simulink model "mech_fceng1"  (Simulink 7.1)
settings: Solver=ode45  StartTime=0.0  StopTime=inf  RelTol=1e-3  AbsTol=1e-4
PreLoadFcn:
  | mech_fceng_init;load mech_fceng_images;
InitFcn:
  | mech_slider_open(gcs);
values from neighbouring files (symbols this model uses):
  AirRo = 1.2E-3    (= 0.0012)    [mech_sceng_init.m]
  Cv = 3    [mech_sceng_init.m]
  G = 9.81    [mech_motorcycle_data.m]    (also in mech_sceng_init.m = 1.4)
  Pa = 1033.34    [mech_sceng_init.m]
  Q = 46816    [mech_sceng_init.m]
  R = y([30:p],2)./y([30:p],1)    [mech_car_handling_sweep.m]    (also in mech_flexible_beamelement.m = [1  0  0; mech_sceng_init.m = 5; mech_toroid_setup.m = 10)
  Ta = 25    [mech_sceng_init.m]
  Vo = pi*R*R*14    (= 1099.55742876)    [mech_sceng_init.m]
  Vtdc = pi*R*R*2    (= 157.079632679)    [mech_sceng_init.m]
libraries: mblibv1 x47, simulink x3, simulink_extras x1
(part 1 of 2)
settings Model: Creator=The MathWorks Inc.  LastModifiedBy=Administrator  ExtModeAutoUpdateStatusClock=off
settings DataIOCC: SignalLoggingName=sigsOut
settings OptimizationCC: BooleanDataType=off  InlineInvariantSignals=on  BufferReusableBoundary=off
settings DebuggingCC: SaveWithParameterizedLinksMsg=none  CheckExecutionContextPreStartOutputMsg=on  CheckExecutionContextRuntimeOutputMsg=on  SignalResolutionControl=TryResolveAllWithWarning  SolverPrmCheckMsg=none  MultiTaskDSMMsg=warning  MultiTaskCondExecSysMsg=none  SigSpecEnsureSampleTimeMsg=none  UnconnectedInputMsg=none  UnconnectedOutputMsg=none  UnconnectedLineMsg=none  StrictBusMsg=None
settings HardwareCC: ProdHWDeviceType=Specified  TargetEndianess=LittleEndian  TargetHWDeviceType=MATLAB Host  ProdEqTarget=off
settings RTWCC: SystemTargetFile=rsim.tlc  TemplateMakefile=rsim_default_tmf  Description=Rapid Simulation Target  ProcessScript=rsim_make_rtw_hook  IncludeERTFirstTime=on
settings RSimTargetCC: TargetFcnLib=ansi_tfl_tmw.mat  TargetFunctionLibrary=ANSI_C  IsPILTarget=off  EnableShiftOperators=on  PortableWordSizes=off
settings SimMechanicsCC: WarnOnRedundantConstraints=off

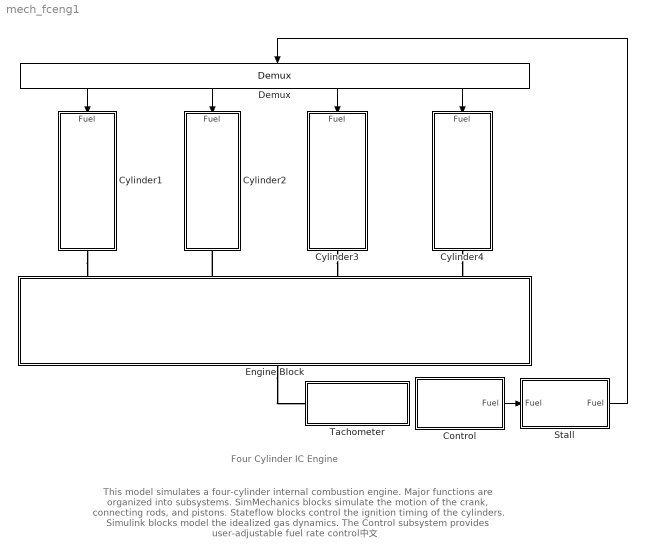
== system mech_fceng1 ==
  note: This model simulates a four-cylinder internal combustion engine. Major functions are organized into subsystems. SimMechanics blocks simulate the motion of the crank, connecting rods, and pistons. Stateflow blocks control the ignition timing of the cylinders. Simulink blocks model the idealized gas dynamics. The Control subsystem provides user-adjustable fuel rate control.中文
  note: Four Cylinder IC Engine
  Control : Subsystem  Tag=OpenMeAtStartUp
  Cylinder1 : Subsystem  Orientation=down
      mask Display: image(crodassm);
  Cylinder2 : Subsystem  Orientation=down
      mask Display: image(crodassmb);
  Cylinder3 : Subsystem  Orientation=down
      mask Display: image(crodassmb);
  Cylinder4 : Subsystem  Orientation=down
      mask Display: image(crodassm);
  Demux : Demux  Orientation=down
  Engine Block : Subsystem  Orientation=up
      mask Display: image(crank);
  Stall : Subsystem
  Tachometer : Subsystem
  wires:
  Demux/1 -> Cylinder1/1(Fuel)
  Demux/2 -> Cylinder2/1(Fuel)
  Demux/3 -> Cylinder3/1(Fuel)
  Demux/4 -> Cylinder4/1(Fuel)
  Control/1(Fuel) -> Stall/1("Fuel ")
  Stall/1(Fuel) -> Demux/1
  connections:
  Cylinder1/RConn1 -- Engine Block/RConn1
  Cylinder4/RConn1 -- Engine Block/RConn4
  Engine Block/LConn1 -- Tachometer/LConn1
  Cylinder3/RConn1 -- Engine Block/RConn3
  Engine Block/RConn2 -- Cylinder2/RConn1

== system mech_fceng1/Control ==
  Constant : Constant  OutDataType=sfix(16)  OutScaling=2^0
  Cylinder1 : simulink/Signal Routing/Manual Switch  Orientation=down  SystemSampleTime=-1  sw=0  action=0  varsize=off
  Cylinder4 : simulink/Signal Routing/Manual Switch  Orientation=down  SystemSampleTime=-1  sw=0  action=0  varsize=off
  Fuel Control : simulink/Math Operations/Slider Gain  Tag="674   438   332   100"  SystemSampleTime=-1  low=0  gain=2  high=4
  OFF : Constant  Orientation=up  Value=0  OutDataType=sfix(16)  OutScaling=2^0
  ON : Constant  Orientation=up  Value=-1  OutDataType=sfix(16)  OutScaling=2^0
  Fuel : Outport  OutDataType=sfix(16)  OutScaling=2^0
  tag scope: Cylinder1=global, Cylinder2=global
  wires:
  Cylinder1/1 -> [Cylinder1]
  Constant/1 -> Fuel Control/1
  Fuel Control/1 -> Fuel/1
  OFF/1 -> Cylinder1/1, Cylinder4/1
  ON/1 -> Cylinder4/2, Cylinder1/2
  Cylinder4/1 -> [Cylinder2]

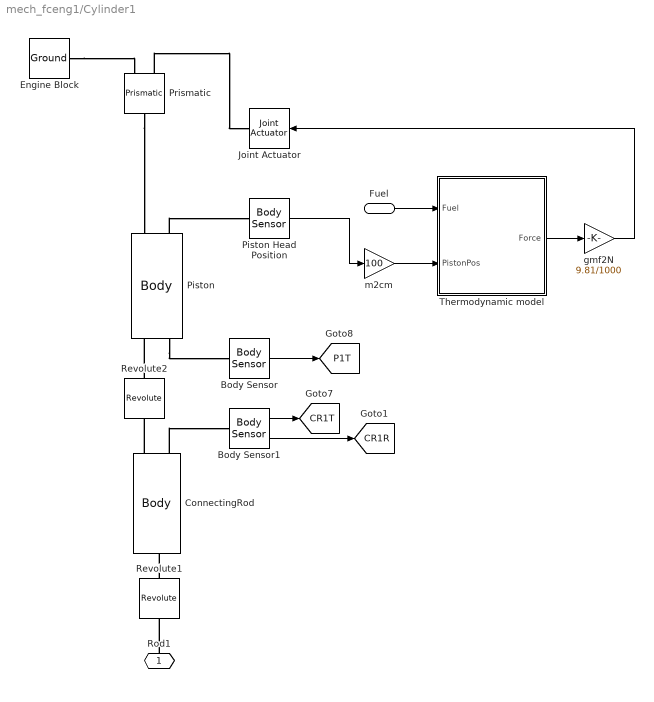
== system mech_fceng1/Cylinder1 ==
  Fuel : Inport  OutDataType=sfix(16)  OutScaling=2^0
  Body Sensor : mblibv1/Sensors &  Actuators/Body Sensor  DialogController=MECH.DynMechDlgSource  SystemSampleTime=-1  PhysicalDomain=Mechanical  PortType=blob  Muxed=on  Pose=off  Angle=on  AngleUnits=deg  ArcVelocity=off  ArcVelocityUnits=deg/s  ArcAcceleration=off  ArcAccelerationUnits=deg/s^2  CoordPosition=on  CoordPositionUnits=m  Velocity=off  VelocityUnits=m/s  Acceleration=off  AccelerationUnits=m/s^2  Quaternion=on  QuaternionDT=off  QuaternionDDT=off  QuaternionUnits=off  OutputVector=[1]  ActiveIO=on  Width=3  DialogClass=MechanicalSensorBlock  ReferenceFrame=Absolute (World)
  Body Sensor1 : mblibv1/Sensors &  Actuators/Body Sensor  DialogController=MECH.DynMechDlgSource  SystemSampleTime=-1  PhysicalDomain=Mechanical  PortType=blob  Muxed=off  Pose=on  Angle=on  AngleUnits=deg  ArcVelocity=off  ArcVelocityUnits=deg/s  ArcAcceleration=off  ArcAccelerationUnits=deg/s^2  CoordPosition=on  CoordPositionUnits=m  Velocity=off  VelocityUnits=m/s  Acceleration=off  AccelerationUnits=m/s^2  Quaternion=on  QuaternionDT=off  QuaternionDDT=off  QuaternionUnits=off  OutputVector=[ 3 9 ]  ActiveIO=on  Width=12  DialogClass=MechanicalSensorBlock  ReferenceFrame=Absolute (World)
  ConnectingRod : mblibv1/Bodies/Body  Orientation=up  DialogController=MECH.DynMechDlgSource  PhysicalDomain=mechanical  SubClassName=Unknown  LeftPortType=workingframe  RightPortType=workingframe  LConnTagsString=CS1  RConnTagsString=CS2|CS3  DialogClass=MechanicalBodyBlock  Mass=676.73  MassUnits=g  InertiaUnits=kg*m^2  Inertia=[37007.64 0 -0.01;0 2936.99 7181.27;-0.01 7181.27 34460.53]*1E-7  Shape=Cylinder  ShapeDims=[1 1]  ShapeUnits=m  ShapeUse=false  Density=1  DensityUnits=kg/m^3  DensityUse=false  GraphicsMode=1  BodyColor=[0.5 0.5 0.5]  GraphicsObj=[]  AttachedToCS=1  CG=Left$CG$[-18 11.35 -2.70]$WORLD$WORLD$cm$[0 0 0]$Euler X-Y-Z$deg$WORLD$false  WorkingFrames=Left$CS1$[-18 4.24 -4.24]$WORLD$WORLD$cm$[0 0 0]$Euler X-Y-Z$deg$WORLD$true#Right$CS2$[-18 23.79 0]$WORLD$WORLD$cm$[0 0 0]$Euler X-Y-Z$deg$WORLD$true#Right$CS3$[-18 4.24 -4.24]$WORLD$WORLD$cm$[0 0 0]$Euler X-Y-Z$deg$WORLD$true  CGPos=[-18 11.35 -2.70]  CGRot=[0 0 0]  CS0Pos=[]  CS0Rot=[]  CS1Pos=[-18 4.24 -4.24]  CS1Rot=[0 0 0]  CS2Pos=[-18 23.79 0]  CS2Rot=[0 0 0]  CS3Pos=[-18 4.24 -4.24]  CS3Rot=[0 0 0]  CS4Pos=[]  CS4Rot=[]  CS5Pos=[]  CS5Rot=[]  CS6Pos=[]  CS6Rot=[]  CS7Pos=[]  CS7Rot=[]  CS8Pos=[]  CS8Rot=[]  CS9Pos=[]  CS9Rot=[]  CS10Pos=[]  CS10Rot=[]  CS11Pos=[]  CS11Rot=[]  CS12Pos=[]  CS12Rot=[]  CS13Pos=[]  CS13Rot=[]  CS14Pos=[]  CS14Rot=[]  CS15Pos=[]  CS15Rot=[]  CS16Pos=[]  CS16Rot=[]  CS17Pos=[]  CS17Rot=[]  CS18Pos=[]  CS18Rot=[]  CS19Pos=[]  CS19Rot=[]  CS20Pos=[]  CS20Rot=[]
  Engine Block : mblibv1/Bodies/Ground  DialogController=MECH.DynMechDlgSource  SystemSampleTime=-1  LeftPortType=env  RightPortType=workingframe  PhysicalDomain=Mechanical  DialogClass=GroundBlock  CoordPosition=[-13.23 23.79 0]  CoordPositionUnits=cm  StateVectorMgrId=-1  MachineId=[0 0]  ShowEnvPort=off
  Joint Actuator : mblibv1/Sensors &  Actuators/Joint Actuator  Orientation=left  DialogController=MECH.DynMechDlgSource  SystemSampleTime=-1  PhysicalDomain=Mechanical  PortType=blob  ActuationStyle=Force  AngleUnits=deg  ArcVelocityUnits=deg/s  ArcAccelerationUnits=deg/s^2  CoordPositionUnits=m  VelocityUnits=m/s  AccelerationUnits=m/s^2  ForceUnits=N  TorqueUnits=N-m  ActiveIO=on  Width=1  DialogClass=MechanicalActuatorBlock  Primitive=P1  ReferenceFrame=Absolute (INERTIAL)
  Piston : mblibv1/Bodies/Body  Orientation=up  DialogController=MECH.DynMechDlgSource  PhysicalDomain=mechanical  SubClassName=Unknown  LeftPortType=workingframe  RightPortType=workingframe  LConnTagsString=CS1|CS3  RConnTagsString=CS2|CS4  DialogClass=MechanicalBodyBlock  Mass=3490.25  MassUnits=g  InertiaUnits=kg*m^2  Inertia=[39798.30 0.06 -0.01;0.06 49173.25 -0.04;-0.01 -0.04 39108.48]*1E-7  Shape=Cylinder  ShapeDims=[1 1]  ShapeUnits=m  ShapeUse=false  Density=1  DensityUnits=kg/m^3  DensityUse=false  GraphicsMode=1  BodyColor=[0.5 0.5 0.5]  GraphicsObj=[]  AttachedToCS=1  CG=Left$CG$[-18 24.51 0]$WORLD$WORLD$cm$[0 0 0]$Euler X-Y-Z$deg$WORLD$false  WorkingFrames=Left$CS1$[-18 23.79 0]$WORLD$WORLD$cm$[0 0 0]$Euler X-Y-Z$deg$WORLD$true#Right$CS2$[-13.23 23.79 0]$WORLD$WORLD$cm$[0 0 0]$Euler X-Y-Z$deg$WORLD$true#Left$CS3$[-18 23.79 0]$WORLD$WORLD$cm$[0 0 0]$Euler X-Y-Z$deg$WORLD$true#Right$CS4$[-18 23.79+4 0]$WORLD$WORLD$cm$[0 0 0]$Euler X-Y-Z$deg$WORLD$true  CGPos=[-18 24.51 0]  CGRot=[0 0 0]  CS0Pos=[]  CS0Rot=[]  CS1Pos=[-18 23.79 0]  CS1Rot=[0 0 0]  CS2Pos=[-13.23 23.79 0]  CS2Rot=[0 0 0]  CS3Pos=[-18 23.79 0]  CS3Rot=[0 0 0]  CS4Pos=[-18 23.79+4 0]  CS4Rot=[0 0 0]  CS5Pos=[]  CS5Rot=[]  CS6Pos=[]  CS6Rot=[]  CS7Pos=[]  CS7Rot=[]  CS8Pos=[]  CS8Rot=[]  CS9Pos=[]  CS9Rot=[]  CS10Pos=[]  CS10Rot=[]  CS11Pos=[]  CS11Rot=[]  CS12Pos=[]  CS12Rot=[]  CS13Pos=[]  CS13Rot=[]  CS14Pos=[]  CS14Rot=[]  CS15Pos=[]  CS15Rot=[]  CS16Pos=[]  CS16Rot=[]  CS17Pos=[]  CS17Rot=[]  CS18Pos=[]  CS18Rot=[]  CS19Pos=[]  CS19Rot=[]  CS20Pos=[]  CS20Rot=[]
  Piston Head Position : mblibv1/Sensors &  Actuators/Body Sensor  DialogController=MECH.DynMechDlgSource  SystemSampleTime=-1  PhysicalDomain=Mechanical  PortType=blob  Muxed=on  Pose=off  Angle=on  AngleUnits=deg  ArcVelocity=off  ArcVelocityUnits=deg/s  ArcAcceleration=off  ArcAccelerationUnits=deg/s^2  CoordPosition=on  CoordPositionUnits=m  Velocity=off  VelocityUnits=m/s  Acceleration=off  AccelerationUnits=m/s^2  Quaternion=on  QuaternionDT=off  QuaternionDDT=off  QuaternionUnits=off  OutputVector=[1]  ActiveIO=on  Width=3  DialogClass=MechanicalSensorBlock  ReferenceFrame=Absolute (World)
  Prismatic : mblibv1/Joints/Prismatic  Orientation=down  DialogController=MECH.DynMechDlgSource  PhysicalDomain=mechanical  SubClassName=Unknown  LeftPortType=blob  RightPortType=blob  LConnTagsString=__newl0|SA1  RConnTagsString=__newr0  NumSAPorts=1  CutJoint=off  MarkAsCut=off  Primitives=prismatic  PrimitiveProps=P1$WORLD$[0 1 0]$prismatic  DialogClass=JointBlock  P1Axis=[0 1 0]
  Revolute1 : mblibv1/Joints/Revolute  Orientation=up  DialogController=MECH.DynMechDlgSource  PhysicalDomain=mechanical  SubClassName=Unknown  LeftPortType=blob  RightPortType=blob  LConnTagsString=__newl0  RConnTagsString=__newr0  NumSAPorts=0  CutJoint=off  MarkAsCut=off  Primitives=revolute  PrimitiveProps=R1$WORLD$[1 0 0]$revolute  DialogClass=JointBlock  R1Axis=[1 0 0]
  Revolute2 : mblibv1/Joints/Revolute  Orientation=up  DialogController=MECH.DynMechDlgSource  PhysicalDomain=mechanical  SubClassName=Unknown  LeftPortType=blob  RightPortType=blob  LConnTagsString=__newl0  RConnTagsString=__newr0  NumSAPorts=0  CutJoint=on  MarkAsCut=off  Primitives=revolute  PrimitiveProps=R1$WORLD$[1 0 0]$revolute  DialogClass=JointBlock  R1Axis=[1 0 0]
  Thermodynamic model : Subsystem
  gmf2N : Gain  Gain=9.81/1000  ParameterDataType=sfix(16)  ParameterScaling=2^0  OutDataType=sfix(16)  OutScaling=2^0  SaturateOnIntegerOverflow=on  OutDataTypeStr=Inherit: Same as input  ParamDataTypeStr=Inherit: Same as input
  m2cm : Gain  Gain=100  ParameterDataType=sfix(16)  ParameterScaling=2^0  OutDataType=sfix(16)  OutScaling=2^0  SaturateOnIntegerOverflow=on  OutDataTypeStr=Inherit: Same as input  ParamDataTypeStr=Inherit: Same as input
  Rod1 : PMIOPort  Orientation=up  Port=1  Side=Right
  tag scope: CR1R=global, CR1T=global, P1T=global
  wires:
  Body Sensor1/2 -> [CR1R]
  Body Sensor1/1 -> [CR1T]
  Body Sensor/1 -> [P1T]
  gmf2N/1 -> Joint Actuator/1
  Fuel/1 -> Thermodynamic model/1(Fuel)
  Piston Head Position/1 -> m2cm/1
  Thermodynamic model/1(Force) -> gmf2N/1
  m2cm/1 -> Thermodynamic model/2(PistonPos)
  connections:
  Prismatic/LConn2 -- Joint Actuator/RConn1
  Prismatic/RConn1 -- Piston/RConn1
  Engine Block/RConn1 -- Prismatic/LConn1
  ConnectingRod/RConn2 -- Body Sensor1/LConn1
  Piston/LConn2 -- Body Sensor/LConn1
  Piston/RConn2 -- Piston Head Position/LConn1
  Rod1/RConn1 -- Revolute1/LConn1
  Revolute2/RConn1 -- Piston/LConn1
  ConnectingRod/RConn1 -- Revolute2/LConn1
  Revolute1/RConn1 -- ConnectingRod/LConn1

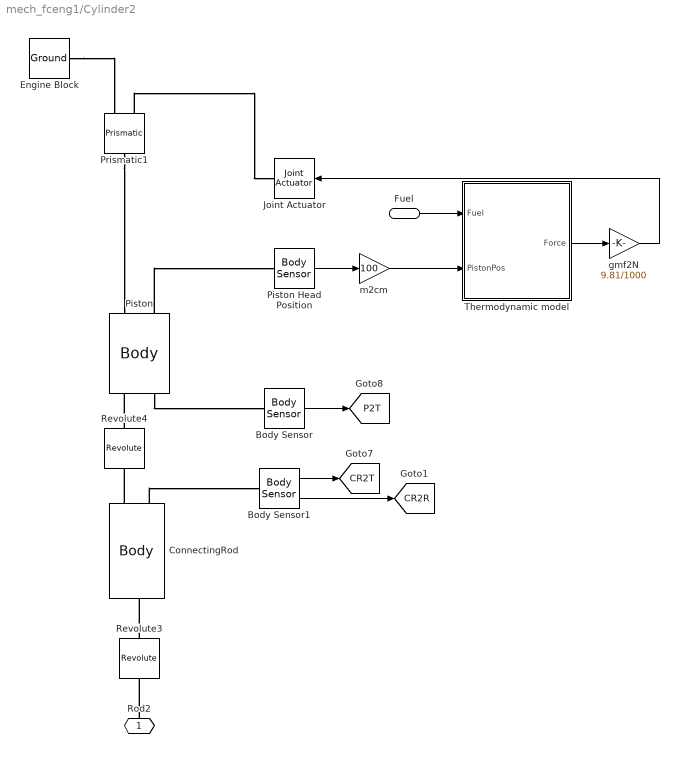
== system mech_fceng1/Cylinder2 ==
  Fuel : Inport  OutDataType=sfix(16)  OutScaling=2^0
  Body Sensor : mblibv1/Sensors &  Actuators/Body Sensor  DialogController=MECH.DynMechDlgSource  SystemSampleTime=-1  PhysicalDomain=Mechanical  PortType=blob  Muxed=on  Pose=off  Angle=on  AngleUnits=deg  ArcVelocity=off  ArcVelocityUnits=deg/s  ArcAcceleration=off  ArcAccelerationUnits=deg/s^2  CoordPosition=on  CoordPositionUnits=m  Velocity=off  VelocityUnits=m/s  Acceleration=off  AccelerationUnits=m/s^2  Quaternion=on  QuaternionDT=off  QuaternionDDT=off  QuaternionUnits=off  OutputVector=[1]  ActiveIO=on  Width=3  DialogClass=MechanicalSensorBlock  ReferenceFrame=Absolute (World)
  Body Sensor1 : mblibv1/Sensors &  Actuators/Body Sensor  DialogController=MECH.DynMechDlgSource  SystemSampleTime=-1  PhysicalDomain=Mechanical  PortType=blob  Muxed=off  Pose=on  Angle=on  AngleUnits=deg  ArcVelocity=off  ArcVelocityUnits=deg/s  ArcAcceleration=off  ArcAccelerationUnits=deg/s^2  CoordPosition=on  CoordPositionUnits=m  Velocity=off  VelocityUnits=m/s  Acceleration=off  AccelerationUnits=m/s^2  Quaternion=on  QuaternionDT=off  QuaternionDDT=off  QuaternionUnits=off  OutputVector=[ 3 9 ]  ActiveIO=on  Width=12  DialogClass=MechanicalSensorBlock  ReferenceFrame=Absolute (World)
  ConnectingRod : mblibv1/Bodies/Body  Orientation=up  DialogController=MECH.DynMechDlgSource  PhysicalDomain=mechanical  SubClassName=Unknown  LeftPortType=workingframe  RightPortType=workingframe  LConnTagsString=CS1  RConnTagsString=CS2|CS3  DialogClass=MechanicalBodyBlock  Mass=676.73  MassUnits=g  InertiaUnits=kg*m^2  Inertia=[37007.64 0 -0.01;0 2936.99 7181.27;-0.01 7181.27 34460.53]*1E-7  Shape=Cylinder  ShapeDims=[1 1]  ShapeUnits=m  ShapeUse=false  Density=1  DensityUnits=kg/m^3  DensityUse=false  GraphicsMode=1  BodyColor=[0.5 0.5 0.5]  GraphicsObj=[]  AttachedToCS=1  CG=Left$CG$[-6 2.87 2.70]$WORLD$WORLD$cm$[0 0 0]$Euler X-Y-Z$deg$WORLD$false  WorkingFrames=Left$CS1$[-6 -4.24 4.24]$WORLD$WORLD$cm$[0 0 0]$Euler X-Y-Z$deg$WORLD$true#Right$CS2$[-6 15.30 0]$WORLD$WORLD$cm$[0 0 0]$Euler X-Y-Z$deg$WORLD$true#Right$CS3$[-6 -4.24 4.24]$WORLD$WORLD$cm$[0 0 0]$Euler X-Y-Z$deg$WORLD$true  CGPos=[-6 2.87 2.70]  CGRot=[0 0 0]  CS0Pos=[]  CS0Rot=[]  CS1Pos=[-6 -4.24 4.24]  CS1Rot=[0 0 0]  CS2Pos=[-6 15.30 0]  CS2Rot=[0 0 0]  CS3Pos=[-6 -4.24 4.24]  CS3Rot=[0 0 0]  CS4Pos=[]  CS4Rot=[]  CS5Pos=[]  CS5Rot=[]  CS6Pos=[]  CS6Rot=[]  CS7Pos=[]  CS7Rot=[]  CS8Pos=[]  CS8Rot=[]  CS9Pos=[]  CS9Rot=[]  CS10Pos=[]  CS10Rot=[]  CS11Pos=[]  CS11Rot=[]  CS12Pos=[]  CS12Rot=[]  CS13Pos=[]  CS13Rot=[]  CS14Pos=[]  CS14Rot=[]  CS15Pos=[]  CS15Rot=[]  CS16Pos=[]  CS16Rot=[]  CS17Pos=[]  CS17Rot=[]  CS18Pos=[]  CS18Rot=[]  CS19Pos=[]  CS19Rot=[]  CS20Pos=[]  CS20Rot=[]
  Engine Block : mblibv1/Bodies/Ground  DialogController=MECH.DynMechDlgSource  SystemSampleTime=-1  LeftPortType=env  RightPortType=workingframe  PhysicalDomain=Mechanical  DialogClass=GroundBlock  CoordPosition=[-1 15.30 0]  CoordPositionUnits=cm  StateVectorMgrId=-1  MachineId=[0 0]  ShowEnvPort=off
  Joint Actuator : mblibv1/Sensors &  Actuators/Joint Actuator  Orientation=left  DialogController=MECH.DynMechDlgSource  SystemSampleTime=-1  PhysicalDomain=Mechanical  PortType=blob  ActuationStyle=Force  AngleUnits=deg  ArcVelocityUnits=deg/s  ArcAccelerationUnits=deg/s^2  CoordPositionUnits=m  VelocityUnits=m/s  AccelerationUnits=m/s^2  ForceUnits=N  TorqueUnits=N-m  ActiveIO=on  Width=1  DialogClass=MechanicalActuatorBlock  Primitive=P1  ReferenceFrame=Absolute (INERTIAL)
  Piston : mblibv1/Bodies/Body  Orientation=up  DialogController=MECH.DynMechDlgSource  PhysicalDomain=mechanical  SubClassName=Unknown  LeftPortType=workingframe  RightPortType=workingframe  LConnTagsString=CS1|CS3  RConnTagsString=CS2|CS4  DialogClass=MechanicalBodyBlock  Mass=3490.25  MassUnits=g  InertiaUnits=kg*m^2  Inertia=[39798.30 0.06 -0.01;0.06 49173.25 -0.04;-0.01 -0.04 39108.48]*1E-7  Shape=Cylinder  ShapeDims=[1 1]  ShapeUnits=m  ShapeUse=false  Density=1  DensityUnits=kg/m^3  DensityUse=false  GraphicsMode=1  BodyColor=[0.5 0.5 0.5]  GraphicsObj=[]  AttachedToCS=1  CG=Left$CG$[-6 16.02 0]$WORLD$WORLD$cm$[0 0 0]$Euler X-Y-Z$deg$WORLD$false  WorkingFrames=Left$CS1$[-6 15.30 0]$WORLD$WORLD$cm$[0 0 0]$Euler X-Y-Z$deg$WORLD$true#Right$CS2$[-1 15.30 0]$WORLD$WORLD$cm$[0 0 0]$Euler X-Y-Z$deg$WORLD$true#Left$CS3$[-6 15.30 0]$WORLD$WORLD$cm$[0 0 0]$Euler X-Y-Z$deg$WORLD$true#Right$CS4$[-6 19.30 0]$WORLD$WORLD$cm$[0 0 0]$Euler X-Y-Z$deg$WORLD$true  CGPos=[-6 16.02 0]  CGRot=[0 0 0]  CS0Pos=[]  CS0Rot=[]  CS1Pos=[-6 15.30 0]  CS1Rot=[0 0 0]  CS2Pos=[-1 15.30 0]  CS2Rot=[0 0 0]  CS3Pos=[-6 15.30 0]  CS3Rot=[0 0 0]  CS4Pos=[-6 19.30 0]  CS4Rot=[0 0 0]  CS5Pos=[]  CS5Rot=[]  CS6Pos=[]  CS6Rot=[]  CS7Pos=[]  CS7Rot=[]  CS8Pos=[]  CS8Rot=[]  CS9Pos=[]  CS9Rot=[]  CS10Pos=[]  CS10Rot=[]  CS11Pos=[]  CS11Rot=[]  CS12Pos=[]  CS12Rot=[]  CS13Pos=[]  CS13Rot=[]  CS14Pos=[]  CS14Rot=[]  CS15Pos=[]  CS15Rot=[]  CS16Pos=[]  CS16Rot=[]  CS17Pos=[]  CS17Rot=[]  CS18Pos=[]  CS18Rot=[]  CS19Pos=[]  CS19Rot=[]  CS20Pos=[]  CS20Rot=[]
  Piston Head Position : mblibv1/Sensors &  Actuators/Body Sensor  DialogController=MECH.DynMechDlgSource  SystemSampleTime=-1  PhysicalDomain=Mechanical  PortType=blob  Muxed=on  Pose=off  Angle=on  AngleUnits=deg  ArcVelocity=off  ArcVelocityUnits=deg/s  ArcAcceleration=off  ArcAccelerationUnits=deg/s^2  CoordPosition=on  CoordPositionUnits=m  Velocity=off  VelocityUnits=m/s  Acceleration=off  AccelerationUnits=m/s^2  Quaternion=on  QuaternionDT=off  QuaternionDDT=off  QuaternionUnits=off  OutputVector=[1]  ActiveIO=on  Width=3  DialogClass=MechanicalSensorBlock  ReferenceFrame=Absolute (World)
  Prismatic1 : mblibv1/Joints/Prismatic  Orientation=down  DialogController=MECH.DynMechDlgSource  PhysicalDomain=mechanical  SubClassName=Unknown  LeftPortType=blob  RightPortType=blob  LConnTagsString=__newl0|SA1  RConnTagsString=__newr0  NumSAPorts=1  CutJoint=off  MarkAsCut=off  Primitives=prismatic  PrimitiveProps=P1$WORLD$[0 1 0]$prismatic  DialogClass=JointBlock  P1Axis=[0 1 0]
  Revolute3 : mblibv1/Joints/Revolute  Orientation=up  DialogController=MECH.DynMechDlgSource  PhysicalDomain=mechanical  SubClassName=Unknown  LeftPortType=blob  RightPortType=blob  LConnTagsString=__newl0  RConnTagsString=__newr0  NumSAPorts=0  CutJoint=off  MarkAsCut=off  Primitives=revolute  PrimitiveProps=R1$WORLD$[1 0 0]$revolute  DialogClass=JointBlock  R1Axis=[1 0 0]
  Revolute4 : mblibv1/Joints/Revolute  Orientation=up  DialogController=MECH.DynMechDlgSource  PhysicalDomain=mechanical  SubClassName=Unknown  LeftPortType=blob  RightPortType=blob  LConnTagsString=__newl0  RConnTagsString=__newr0  NumSAPorts=0  CutJoint=on  MarkAsCut=off  Primitives=revolute  PrimitiveProps=R1$WORLD$[1 0 0]$revolute  DialogClass=JointBlock  R1Axis=[1 0 0]
  Thermodynamic model : Subsystem
  gmf2N : Gain  Gain=9.81/1000  ParameterDataType=sfix(16)  ParameterScaling=2^0  OutDataType=sfix(16)  OutScaling=2^0  SaturateOnIntegerOverflow=on  OutDataTypeStr=Inherit: Same as input  ParamDataTypeStr=Inherit: Same as input
  m2cm : Gain  Gain=100  ParameterDataType=sfix(16)  ParameterScaling=2^0  OutDataType=sfix(16)  OutScaling=2^0  SaturateOnIntegerOverflow=on  OutDataTypeStr=Inherit: Same as input  ParamDataTypeStr=Inherit: Same as input
  Rod2 : PMIOPort  Orientation=up  Port=1  Side=Right
  tag scope: CR2R=global, CR2T=global, P2T=global
  wires:
  Body Sensor1/2 -> [CR2R]
  Body Sensor/1 -> [P2T]
  Body Sensor1/1 -> [CR2T]
  gmf2N/1 -> Joint Actuator/1
  Fuel/1 -> Thermodynamic model/1(Fuel)
  Piston Head Position/1 -> m2cm/1
  Thermodynamic model/1(Force) -> gmf2N/1
  m2cm/1 -> Thermodynamic model/2(PistonPos)
  connections:
  Prismatic1/LConn2 -- Joint Actuator/RConn1
  Prismatic1/RConn1 -- Piston/RConn1
  Engine Block/RConn1 -- Prismatic1/LConn1
  ConnectingRod/RConn2 -- Body Sensor1/LConn1
  Piston/LConn2 -- Body Sensor/LConn1
  Piston/RConn2 -- Piston Head Position/LConn1
  Revolute3/RConn1 -- ConnectingRod/LConn1
  ConnectingRod/RConn1 -- Revolute4/LConn1
  Revolute4/RConn1 -- Piston/LConn1
  Rod2/RConn1 -- Revolute3/LConn1

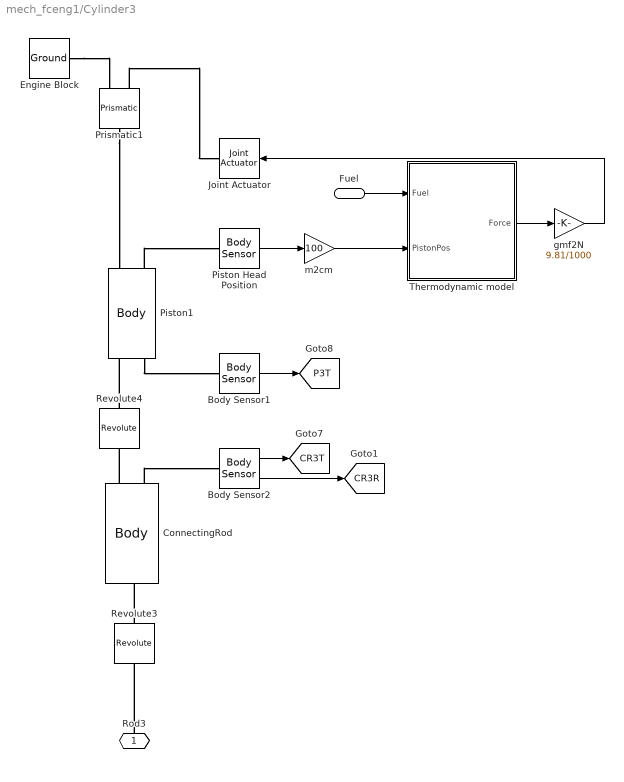
== system mech_fceng1/Cylinder3 ==
  Fuel : Inport  OutDataType=sfix(16)  OutScaling=2^0
  Body Sensor1 : mblibv1/Sensors &  Actuators/Body Sensor  DialogController=MECH.DynMechDlgSource  SystemSampleTime=-1  PhysicalDomain=Mechanical  PortType=blob  Muxed=on  Pose=off  Angle=on  AngleUnits=deg  ArcVelocity=off  ArcVelocityUnits=deg/s  ArcAcceleration=off  ArcAccelerationUnits=deg/s^2  CoordPosition=on  CoordPositionUnits=m  Velocity=off  VelocityUnits=m/s  Acceleration=off  AccelerationUnits=m/s^2  Quaternion=on  QuaternionDT=off  QuaternionDDT=off  QuaternionUnits=off  OutputVector=[1]  ActiveIO=on  Width=3  DialogClass=MechanicalSensorBlock  ReferenceFrame=Absolute (World)
  Body Sensor2 : mblibv1/Sensors &  Actuators/Body Sensor  DialogController=MECH.DynMechDlgSource  SystemSampleTime=-1  PhysicalDomain=Mechanical  PortType=blob  Muxed=off  Pose=on  Angle=on  AngleUnits=deg  ArcVelocity=off  ArcVelocityUnits=deg/s  ArcAcceleration=off  ArcAccelerationUnits=deg/s^2  CoordPosition=on  CoordPositionUnits=m  Velocity=off  VelocityUnits=m/s  Acceleration=off  AccelerationUnits=m/s^2  Quaternion=on  QuaternionDT=off  QuaternionDDT=off  QuaternionUnits=off  OutputVector=[ 3 9 ]  ActiveIO=on  Width=12  DialogClass=MechanicalSensorBlock  ReferenceFrame=Absolute (World)
  ConnectingRod : mblibv1/Bodies/Body  Orientation=up  DialogController=MECH.DynMechDlgSource  PhysicalDomain=mechanical  SubClassName=Unknown  LeftPortType=workingframe  RightPortType=workingframe  LConnTagsString=CS1  RConnTagsString=CS2|CS3  DialogClass=MechanicalBodyBlock  Mass=676.73  MassUnits=g  InertiaUnits=kg*m^2  Inertia=[37007.64 0 -0.01;0 2936.99 7181.27;-0.01 7181.27 34460.53]*1E-7  Shape=Cylinder  ShapeDims=[1 1]  ShapeUnits=m  ShapeUse=false  Density=1  DensityUnits=kg/m^3  DensityUse=false  GraphicsMode=1  BodyColor=[0.5 0.5 0.5]  GraphicsObj=[]  AttachedToCS=1  CG=Left$CG$[6 2.87 2.70]$WORLD$WORLD$cm$[0 0 0]$Euler X-Y-Z$deg$WORLD$false  WorkingFrames=Left$CS1$[6 -4.24 4.24]$WORLD$WORLD$cm$[0 0 0]$Euler X-Y-Z$deg$WORLD$true#Right$CS2$[6 15.30 0]$WORLD$WORLD$cm$[0 0 0]$Euler X-Y-Z$deg$WORLD$true#Right$CS3$[6 -4.24 4.24]$WORLD$WORLD$cm$[0 0 0]$Euler X-Y-Z$deg$WORLD$true  CGPos=[6 2.87 2.70]  CGRot=[0 0 0]  CS0Pos=[]  CS0Rot=[]  CS1Pos=[6 -4.24 4.24]  CS1Rot=[0 0 0]  CS2Pos=[6 15.30 0]  CS2Rot=[0 0 0]  CS3Pos=[6 -4.24 4.24]  CS3Rot=[0 0 0]  CS4Pos=[]  CS4Rot=[]  CS5Pos=[]  CS5Rot=[]  CS6Pos=[]  CS6Rot=[]  CS7Pos=[]  CS7Rot=[]  CS8Pos=[]  CS8Rot=[]  CS9Pos=[]  CS9Rot=[]  CS10Pos=[]  CS10Rot=[]  CS11Pos=[]  CS11Rot=[]  CS12Pos=[]  CS12Rot=[]  CS13Pos=[]  CS13Rot=[]  CS14Pos=[]  CS14Rot=[]  CS15Pos=[]  CS15Rot=[]  CS16Pos=[]  CS16Rot=[]  CS17Pos=[]  CS17Rot=[]  CS18Pos=[]  CS18Rot=[]  CS19Pos=[]  CS19Rot=[]  CS20Pos=[]  CS20Rot=[]
  Engine Block : mblibv1/Bodies/Ground  DialogController=MECH.DynMechDlgSource  SystemSampleTime=-1  LeftPortType=env  RightPortType=workingframe  PhysicalDomain=Mechanical  DialogClass=GroundBlock  CoordPosition=[11 15.30 0]  CoordPositionUnits=cm  StateVectorMgrId=-1  MachineId=[0 0]  ShowEnvPort=off
  Joint Actuator : mblibv1/Sensors &  Actuators/Joint Actuator  Orientation=left  DialogController=MECH.DynMechDlgSource  SystemSampleTime=-1  PhysicalDomain=Mechanical  PortType=blob  ActuationStyle=Force  AngleUnits=deg  ArcVelocityUnits=deg/s  ArcAccelerationUnits=deg/s^2  CoordPositionUnits=m  VelocityUnits=m/s  AccelerationUnits=m/s^2  ForceUnits=N  TorqueUnits=N-m  ActiveIO=on  Width=1  DialogClass=MechanicalActuatorBlock  Primitive=P1  ReferenceFrame=Absolute (INERTIAL)
  Piston Head Position : mblibv1/Sensors &  Actuators/Body Sensor  DialogController=MECH.DynMechDlgSource  SystemSampleTime=-1  PhysicalDomain=Mechanical  PortType=blob  Muxed=on  Pose=off  Angle=on  AngleUnits=deg  ArcVelocity=off  ArcVelocityUnits=deg/s  ArcAcceleration=off  ArcAccelerationUnits=deg/s^2  CoordPosition=on  CoordPositionUnits=m  Velocity=off  VelocityUnits=m/s  Acceleration=off  AccelerationUnits=m/s^2  Quaternion=on  QuaternionDT=off  QuaternionDDT=off  QuaternionUnits=off  OutputVector=[1]  ActiveIO=on  Width=3  DialogClass=MechanicalSensorBlock  ReferenceFrame=Absolute (World)
  Piston1 : mblibv1/Bodies/Body  Orientation=up  DialogController=MECH.DynMechDlgSource  PhysicalDomain=mechanical  SubClassName=Unknown  LeftPortType=workingframe  RightPortType=workingframe  LConnTagsString=CS1|CS3  RConnTagsString=CS2|CS4  DialogClass=MechanicalBodyBlock  Mass=3490.25  MassUnits=g  InertiaUnits=kg*m^2  Inertia=[39798.30 0.06 -0.01;0.06 49173.25 -0.04;-0.01 -0.04 39108.48]*1E-7  Shape=Cylinder  ShapeDims=[1 1]  ShapeUnits=m  ShapeUse=false  Density=1  DensityUnits=kg/m^3  DensityUse=false  GraphicsMode=1  BodyColor=[0.5 0.5 0.5]  GraphicsObj=[]  AttachedToCS=1  CG=Left$CG$[6 16.02 0]$WORLD$WORLD$cm$[0 0 0]$Euler X-Y-Z$deg$WORLD$false  WorkingFrames=Left$CS1$[6 15.30 0]$WORLD$WORLD$cm$[0 0 0]$Euler X-Y-Z$deg$WORLD$true#Right$CS2$[11 15.30 0]$WORLD$WORLD$cm$[0 0 0]$Euler X-Y-Z$deg$WORLD$true#Left$CS3$[6 15.30 0]$WORLD$WORLD$cm$[0 0 0]$Euler X-Y-Z$deg$WORLD$true#Right$CS4$[6 15.30+4 0]$WORLD$WORLD$cm$[0 0 0]$Euler X-Y-Z$deg$WORLD$true  CGPos=[6 16.02 0]  CGRot=[0 0 0]  CS0Pos=[]  CS0Rot=[]  CS1Pos=[6 15.30 0]  CS1Rot=[0 0 0]  CS2Pos=[11 15.30 0]  CS2Rot=[0 0 0]  CS3Pos=[6 15.30 0]  CS3Rot=[0 0 0]  CS4Pos=[6 15.30+4 0]  CS4Rot=[0 0 0]  CS5Pos=[]  CS5Rot=[]  CS6Pos=[]  CS6Rot=[]  CS7Pos=[]  CS7Rot=[]  CS8Pos=[]  CS8Rot=[]  CS9Pos=[]  CS9Rot=[]  CS10Pos=[]  CS10Rot=[]  CS11Pos=[]  CS11Rot=[]  CS12Pos=[]  CS12Rot=[]  CS13Pos=[]  CS13Rot=[]  CS14Pos=[]  CS14Rot=[]  CS15Pos=[]  CS15Rot=[]  CS16Pos=[]  CS16Rot=[]  CS17Pos=[]  CS17Rot=[]  CS18Pos=[]  CS18Rot=[]  CS19Pos=[]  CS19Rot=[]  CS20Pos=[]  CS20Rot=[]
  Prismatic1 : mblibv1/Joints/Prismatic  Orientation=down  DialogController=MECH.DynMechDlgSource  PhysicalDomain=mechanical  SubClassName=Unknown  LeftPortType=blob  RightPortType=blob  LConnTagsString=__newl0|SA1  RConnTagsString=__newr0  NumSAPorts=1  CutJoint=off  MarkAsCut=off  Primitives=prismatic  PrimitiveProps=P1$WORLD$[0 1 0]$prismatic  DialogClass=JointBlock  P1Axis=[0 1 0]
  Revolute3 : mblibv1/Joints/Revolute  Orientation=up  DialogController=MECH.DynMechDlgSource  PhysicalDomain=mechanical  SubClassName=Unknown  LeftPortType=blob  RightPortType=blob  LConnTagsString=__newl0  RConnTagsString=__newr0  NumSAPorts=0  CutJoint=off  MarkAsCut=off  Primitives=revolute  PrimitiveProps=R1$WORLD$[1 0 0]$revolute  DialogClass=JointBlock  R1Axis=[1 0 0]
  Revolute4 : mblibv1/Joints/Revolute  Orientation=up  DialogController=MECH.DynMechDlgSource  PhysicalDomain=mechanical  SubClassName=Unknown  LeftPortType=blob  RightPortType=blob  LConnTagsString=__newl0  RConnTagsString=__newr0  NumSAPorts=0  CutJoint=on  MarkAsCut=off  Primitives=revolute  PrimitiveProps=R1$WORLD$[1 0 0]$revolute  DialogClass=JointBlock  R1Axis=[1 0 0]
  Thermodynamic model : Subsystem
  gmf2N : Gain  Gain=9.81/1000  ParameterDataType=sfix(16)  ParameterScaling=2^0  OutDataType=sfix(16)  OutScaling=2^0  SaturateOnIntegerOverflow=on  OutDataTypeStr=Inherit: Same as input  ParamDataTypeStr=Inherit: Same as input
  m2cm : Gain  Gain=100  ParameterDataType=sfix(16)  ParameterScaling=2^0  OutDataType=sfix(16)  OutScaling=2^0  SaturateOnIntegerOverflow=on  OutDataTypeStr=Inherit: Same as input  ParamDataTypeStr=Inherit: Same as input
  Rod3 : PMIOPort  Orientation=up  Port=1  Side=Right
  tag scope: CR3R=global, CR3T=global, P3T=global
  wires:
  Body Sensor2/2 -> [CR3R]
  Body Sensor2/1 -> [CR3T]
  Body Sensor1/1 -> [P3T]
  gmf2N/1 -> Joint Actuator/1
  Fuel/1 -> Thermodynamic model/1(Fuel)
  Piston Head Position/1 -> m2cm/1
  Thermodynamic model/1(Force) -> gmf2N/1
  m2cm/1 -> Thermodynamic model/2(PistonPos)
  connections:
  Prismatic1/LConn2 -- Joint Actuator/RConn1
  Prismatic1/RConn1 -- Piston1/RConn1
  Engine Block/RConn1 -- Prismatic1/LConn1
  Piston1/LConn2 -- Body Sensor1/LConn1
  ConnectingRod/RConn2 -- Body Sensor2/LConn1
  Rod3/RConn1 -- Revolute3/LConn1
  Revolute4/RConn1 -- Piston1/LConn1
  ConnectingRod/RConn1 -- Revolute4/LConn1
  Revolute3/RConn1 -- ConnectingRod/LConn1
  Piston1/RConn2 -- Piston Head Position/LConn1

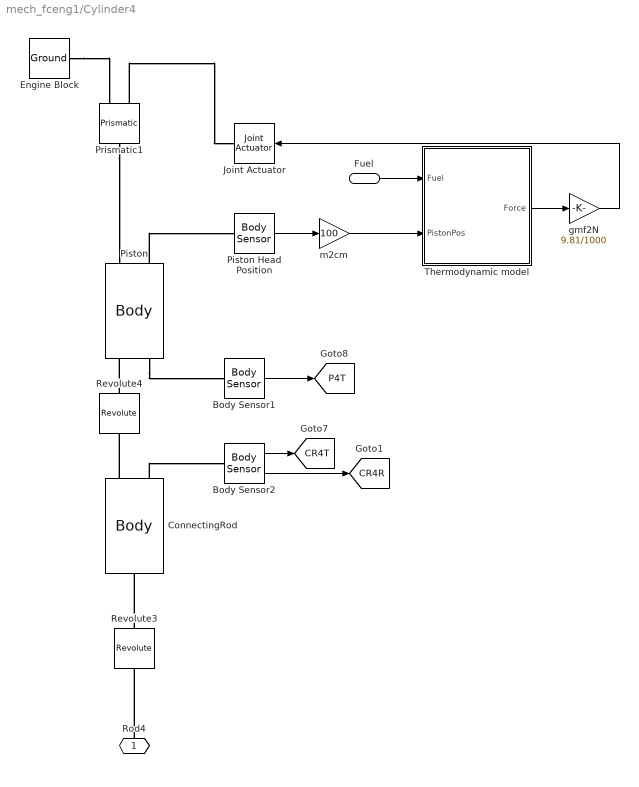
== system mech_fceng1/Cylinder4 ==
  Fuel : Inport  OutDataType=sfix(16)  OutScaling=2^0
  Body Sensor1 : mblibv1/Sensors &  Actuators/Body Sensor  DialogController=MECH.DynMechDlgSource  SystemSampleTime=-1  PhysicalDomain=Mechanical  PortType=blob  Muxed=on  Pose=off  Angle=on  AngleUnits=deg  ArcVelocity=off  ArcVelocityUnits=deg/s  ArcAcceleration=off  ArcAccelerationUnits=deg/s^2  CoordPosition=on  CoordPositionUnits=m  Velocity=off  VelocityUnits=m/s  Acceleration=off  AccelerationUnits=m/s^2  Quaternion=on  QuaternionDT=off  QuaternionDDT=off  QuaternionUnits=off  OutputVector=[1]  ActiveIO=on  Width=3  DialogClass=MechanicalSensorBlock  ReferenceFrame=Absolute (INERTIAL)
  Body Sensor2 : mblibv1/Sensors &  Actuators/Body Sensor  DialogController=MECH.DynMechDlgSource  SystemSampleTime=-1  PhysicalDomain=Mechanical  PortType=blob  Muxed=off  Pose=on  Angle=on  AngleUnits=deg  ArcVelocity=off  ArcVelocityUnits=deg/s  ArcAcceleration=off  ArcAccelerationUnits=deg/s^2  CoordPosition=on  CoordPositionUnits=m  Velocity=off  VelocityUnits=m/s  Acceleration=off  AccelerationUnits=m/s^2  Quaternion=on  QuaternionDT=off  QuaternionDDT=off  QuaternionUnits=off  OutputVector=[ 3 9 ]  ActiveIO=on  Width=12  DialogClass=MechanicalSensorBlock  ReferenceFrame=Absolute (World)
  ConnectingRod : mblibv1/Bodies/Body  Orientation=up  DialogController=MECH.DynMechDlgSource  PhysicalDomain=mechanical  SubClassName=Unknown  LeftPortType=workingframe  RightPortType=workingframe  LConnTagsString=CS1  RConnTagsString=CS2|CS3  DialogClass=MechanicalBodyBlock  Mass=676.73  MassUnits=g  InertiaUnits=kg*m^2  Inertia=[37007.64 0 -0.01;0 2936.99 7181.27;-0.01 7181.27 34460.53]*1E-7  Shape=Cylinder  ShapeDims=[1 1]  ShapeUnits=m  ShapeUse=false  Density=1  DensityUnits=kg/m^3  DensityUse=false  GraphicsMode=1  BodyColor=[0.5 0.5 0.5]  GraphicsObj=[]  AttachedToCS=1  CG=Left$CG$[18 11.35 -2.70]$WORLD$WORLD$cm$[0 0 0]$Euler X-Y-Z$deg$WORLD$false  WorkingFrames=Left$CS1$[18 4.24 -4.24]$WORLD$WORLD$cm$[0 0 0]$Euler X-Y-Z$deg$WORLD$true#Right$CS2$[18 23.79 0]$WORLD$WORLD$cm$[0 0 0]$Euler X-Y-Z$deg$WORLD$true#Right$CS3$[18 4.24 -4.24]$WORLD$WORLD$cm$[0 0 0]$Euler X-Y-Z$deg$WORLD$true  CGPos=[18 11.35 -2.70]  CGRot=[0 0 0]  CS0Pos=[]  CS0Rot=[]  CS1Pos=[18 4.24 -4.24]  CS1Rot=[0 0 0]  CS2Pos=[18 23.79 0]  CS2Rot=[0 0 0]  CS3Pos=[18 4.24 -4.24]  CS3Rot=[0 0 0]  CS4Pos=[]  CS4Rot=[]  CS5Pos=[]  CS5Rot=[]  CS6Pos=[]  CS6Rot=[]  CS7Pos=[]  CS7Rot=[]  CS8Pos=[]  CS8Rot=[]  CS9Pos=[]  CS9Rot=[]  CS10Pos=[]  CS10Rot=[]  CS11Pos=[]  CS11Rot=[]  CS12Pos=[]  CS12Rot=[]  CS13Pos=[]  CS13Rot=[]  CS14Pos=[]  CS14Rot=[]  CS15Pos=[]  CS15Rot=[]  CS16Pos=[]  CS16Rot=[]  CS17Pos=[]  CS17Rot=[]  CS18Pos=[]  CS18Rot=[]  CS19Pos=[]  CS19Rot=[]  CS20Pos=[]  CS20Rot=[]
  Engine Block : mblibv1/Bodies/Ground  DialogController=MECH.DynMechDlgSource  SystemSampleTime=-1  LeftPortType=env  RightPortType=workingframe  PhysicalDomain=Mechanical  DialogClass=GroundBlock  CoordPosition=[23 23.79 0]  CoordPositionUnits=cm  StateVectorMgrId=-1  MachineId=[0 0]  ShowEnvPort=off
  Joint Actuator : mblibv1/Sensors &  Actuators/Joint Actuator  Orientation=left  DialogController=MECH.DynMechDlgSource  SystemSampleTime=-1  PhysicalDomain=Mechanical  PortType=blob  ActuationStyle=Force  AngleUnits=deg  ArcVelocityUnits=deg/s  ArcAccelerationUnits=deg/s^2  CoordPositionUnits=m  VelocityUnits=m/s  AccelerationUnits=m/s^2  ForceUnits=N  TorqueUnits=N-m  ActiveIO=on  Width=1  DialogClass=MechanicalActuatorBlock  Primitive=P1  ReferenceFrame=Absolute (INERTIAL)
  Piston : mblibv1/Bodies/Body  Orientation=up  DialogController=MECH.DynMechDlgSource  PhysicalDomain=mechanical  SubClassName=Unknown  LeftPortType=workingframe  RightPortType=workingframe  LConnTagsString=CS1|CS3  RConnTagsString=CS2|CS4  DialogClass=MechanicalBodyBlock  Mass=3490.25  MassUnits=g  InertiaUnits=kg*m^2  Inertia=[39798.30 0.06 -0.01;0.06 49173.25 -0.04;-0.01 -0.04 39108.48]*1E-7  Shape=Cylinder  ShapeDims=[1 1]  ShapeUnits=m  ShapeUse=false  Density=1  DensityUnits=kg/m^3  DensityUse=false  GraphicsMode=1  BodyColor=[0.5 0.5 0.5]  GraphicsObj=[]  AttachedToCS=1  CG=Left$CG$[18 24.51 0]$WORLD$WORLD$cm$[0 0 0]$Euler X-Y-Z$deg$WORLD$false  WorkingFrames=Left$CS1$[18 23.79 0]$WORLD$WORLD$cm$[0 0 0]$Euler X-Y-Z$deg$WORLD$true#Right$CS2$[23 23.79 0]$WORLD$WORLD$cm$[0 0 0]$Euler X-Y-Z$deg$WORLD$true#Left$CS3$[18 23.79 0]$WORLD$WORLD$cm$[0 0 0]$Euler X-Y-Z$deg$WORLD$true#Right$CS4$[18 23.79+4 0]$WORLD$WORLD$cm$[0 0 0]$Euler X-Y-Z$deg$WORLD$true  CGPos=[18 24.51 0]  CGRot=[0 0 0]  CS0Pos=[]  CS0Rot=[]  CS1Pos=[18 23.79 0]  CS1Rot=[0 0 0]  CS2Pos=[23 23.79 0]  CS2Rot=[0 0 0]  CS3Pos=[18 23.79 0]  CS3Rot=[0 0 0]  CS4Pos=[18 23.79+4 0]  CS4Rot=[0 0 0]  CS5Pos=[]  CS5Rot=[]  CS6Pos=[]  CS6Rot=[]  CS7Pos=[]  CS7Rot=[]  CS8Pos=[]  CS8Rot=[]  CS9Pos=[]  CS9Rot=[]  CS10Pos=[]  CS10Rot=[]  CS11Pos=[]  CS11Rot=[]  CS12Pos=[]  CS12Rot=[]  CS13Pos=[]  CS13Rot=[]  CS14Pos=[]  CS14Rot=[]  CS15Pos=[]  CS15Rot=[]  CS16Pos=[]  CS16Rot=[]  CS17Pos=[]  CS17Rot=[]  CS18Pos=[]  CS18Rot=[]  CS19Pos=[]  CS19Rot=[]  CS20Pos=[]  CS20Rot=[]
  Piston Head Position : mblibv1/Sensors &  Actuators/Body Sensor  DialogController=MECH.DynMechDlgSource  SystemSampleTime=-1  PhysicalDomain=Mechanical  PortType=blob  Muxed=on  Pose=off  Angle=on  AngleUnits=deg  ArcVelocity=off  ArcVelocityUnits=deg/s  ArcAcceleration=off  ArcAccelerationUnits=deg/s^2  CoordPosition=on  CoordPositionUnits=m  Velocity=off  VelocityUnits=m/s  Acceleration=off  AccelerationUnits=m/s^2  Quaternion=on  QuaternionDT=off  QuaternionDDT=off  QuaternionUnits=off  OutputVector=[1]  ActiveIO=on  Width=3  DialogClass=MechanicalSensorBlock  ReferenceFrame=Absolute (World)
  Prismatic1 : mblibv1/Joints/Prismatic  Orientation=down  DialogController=MECH.DynMechDlgSource  PhysicalDomain=mechanical  SubClassName=Unknown  LeftPortType=blob  RightPortType=blob  LConnTagsString=__newl0|SA1  RConnTagsString=__newr0  NumSAPorts=1  CutJoint=off  MarkAsCut=off  Primitives=prismatic  PrimitiveProps=P1$WORLD$[0 1 0]$prismatic  DialogClass=JointBlock  P1Axis=[0 1 0]
  Revolute3 : mblibv1/Joints/Revolute  Orientation=up  DialogController=MECH.DynMechDlgSource  PhysicalDomain=mechanical  SubClassName=Unknown  LeftPortType=blob  RightPortType=blob  LConnTagsString=__newl0  RConnTagsString=__newr0  NumSAPorts=0  CutJoint=off  MarkAsCut=off  Primitives=revolute  PrimitiveProps=R1$WORLD$[1 0 0]$revolute  DialogClass=JointBlock  R1Axis=[1 0 0]
  Revolute4 : mblibv1/Joints/Revolute  Orientation=up  DialogController=MECH.DynMechDlgSource  PhysicalDomain=mechanical  SubClassName=Unknown  LeftPortType=blob  RightPortType=blob  LConnTagsString=__newl0  RConnTagsString=__newr0  NumSAPorts=0  CutJoint=on  MarkAsCut=off  Primitives=revolute  PrimitiveProps=R1$WORLD$[1 0 0]$revolute  DialogClass=JointBlock  R1Axis=[1 0 0]
  Thermodynamic model : Subsystem
  gmf2N : Gain  Gain=9.81/1000  ParameterDataType=sfix(16)  ParameterScaling=2^0  OutDataType=sfix(16)  OutScaling=2^0  SaturateOnIntegerOverflow=on  OutDataTypeStr=Inherit: Same as input  ParamDataTypeStr=Inherit: Same as input
  m2cm : Gain  Gain=100  ParameterDataType=sfix(16)  ParameterScaling=2^0  OutDataType=sfix(16)  OutScaling=2^0  SaturateOnIntegerOverflow=on  OutDataTypeStr=Inherit: Same as input  ParamDataTypeStr=Inherit: Same as input
  Rod4 : PMIOPort  Orientation=up  Port=1  Side=Right
  tag scope: CR4R=global, CR4T=global, P4T=global
  wires:
  Body Sensor2/2 -> [CR4R]
  Body Sensor2/1 -> [CR4T]
  Body Sensor1/1 -> [P4T]
  m2cm/1 -> Thermodynamic model/2(PistonPos)
  Thermodynamic model/1(Force) -> gmf2N/1
  Piston Head Position/1 -> m2cm/1
  Fuel/1 -> Thermodynamic model/1(Fuel)
  gmf2N/1 -> Joint Actuator/1
  connections:
  Prismatic1/LConn2 -- Joint Actuator/RConn1
  Prismatic1/RConn1 -- Piston/RConn1
  Engine Block/RConn1 -- Prismatic1/LConn1
  ConnectingRod/RConn2 -- Body Sensor2/LConn1
  Piston/LConn2 -- Body Sensor1/LConn1
  Piston/RConn2 -- Piston Head Position/LConn1
  Rod4/RConn1 -- Revolute3/LConn1
  Revolute3/RConn1 -- ConnectingRod/LConn1
  ConnectingRod/RConn1 -- Revolute4/LConn1
  Revolute4/RConn1 -- Piston/LConn1

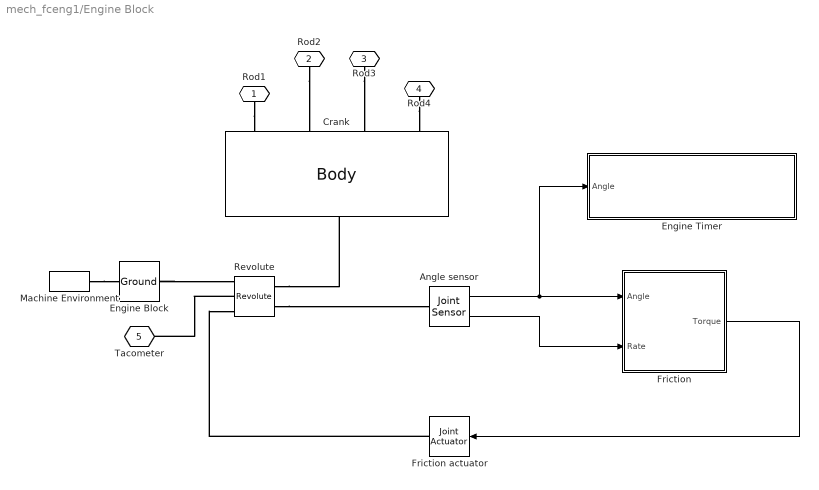
== system mech_fceng1/Engine Block ==
  Angle sensor : mblibv1/Sensors &  Actuators/Joint Sensor  DialogController=MECH.DynMechDlgSource  SystemSampleTime=-1  PhysicalDomain=Mechanical  PortType=blob  Muxed=off  Pose=on  Angle=on  AngleUnits=rad  ArcVelocity=on  ArcVelocityUnits=rad/s  ArcAcceleration=off  ArcAccelerationUnits=deg/s^2  CoordPosition=on  CoordPositionUnits=m  Velocity=off  VelocityUnits=m/s  Acceleration=off  AccelerationUnits=m/s^2  Quaternion=on  QuaternionDT=off  QuaternionDDT=off  QuaternionUnits=off  OutputVector=[ 1 1 ]  ActiveIO=on  Width=2  DialogClass=MechanicalSensorBlock  Primitive=R1  Force=off  ForceUnits=N  Torque=off  TorqueUnits=N-m  ReferenceFrame=Absolute (INERTIAL)  ReactionSensedSide=Base  ReactionReferenceFrame=Absolute (World)  ReactionForce=off  ReactionForceUnits=N  ReactionMoment=off  ReactionMomentUnits=N-m
  Crank : mblibv1/Bodies/Body  Orientation=up  DialogController=MECH.DynMechDlgSource  PhysicalDomain=mechanical  SubClassName=Unknown  LeftPortType=workingframe  RightPortType=workingframe  LConnTagsString=CS1  RConnTagsString=CS2|CS3|CS4|CS5  DialogClass=MechanicalBodyBlock  Mass=33846.54  MassUnits=g  InertiaUnits=kg*m^2  Inertia=[1159762.55 0 0;0 9246514.71 -187767.86;0 -187767.86 9246514.71]*1E-5  Shape=Cylinder  ShapeDims=[1 1]  ShapeUnits=m  ShapeUse=false  Density=1  DensityUnits=kg/m^3  DensityUse=false  GraphicsMode=1  BodyColor=[0.5 0.5 0.5]  GraphicsObj=[]  AttachedToCS=1  CG=Left$CG$[4.45 0 0]$WORLD$WORLD$cm$[0 0 0]$Euler X-Y-Z$deg$WORLD$false  WorkingFrames=Left$CS1$[0 0 0]$WORLD$WORLD$cm$[0 0 0]$Euler X-Y-Z$deg$WORLD$true#Right$CS2$[-18 4.24 -4.24]$WORLD$WORLD$cm$[0 0 0]$Euler X-Y-Z$deg$WORLD$true#Right$CS3$[-6 -4.24 4.24]$WORLD$WORLD$cm$[0 0 0]$Euler X-Y-Z$deg$WORLD$true#Right$CS4$[6 -4.24 4.24]$WORLD$WORLD$cm$[0 0 0]$Euler X-Y-Z$deg$WORLD$true#Right$CS5$[18 4.24 -4.24]$WORLD$WORLD$cm$[0 0 0]$Euler X-Y-Z$deg$WORLD$true  CGPos=[4.45 0 0]  CGRot=[0 0 0]  CS0Pos=[]  CS0Rot=[]  CS1Pos=[0 0 0]  CS1Rot=[0 0 0]  CS2Pos=[-18 4.24 -4.24]  CS2Rot=[0 0 0]  CS3Pos=[-6 -4.24 4.24]  CS3Rot=[0 0 0]  CS4Pos=[6 -4.24 4.24]  CS4Rot=[0 0 0]  CS5Pos=[18 4.24 -4.24]  CS5Rot=[0 0 0]  CS6Pos=[]  CS6Rot=[]  CS7Pos=[]  CS7Rot=[]  CS8Pos=[]  CS8Rot=[]  CS9Pos=[]  CS9Rot=[]  CS10Pos=[]  CS10Rot=[]  CS11Pos=[]  CS11Rot=[]  CS12Pos=[]  CS12Rot=[]  CS13Pos=[]  CS13Rot=[]  CS14Pos=[]  CS14Rot=[]  CS15Pos=[]  CS15Rot=[]  CS16Pos=[]  CS16Rot=[]  CS17Pos=[]  CS17Rot=[]  CS18Pos=[]  CS18Rot=[]  CS19Pos=[]  CS19Rot=[]  CS20Pos=[]  CS20Rot=[]
  Engine Block : mblibv1/Bodies/Ground  DialogController=MECH.DynMechDlgSource  SystemSampleTime=-1  LeftPortType=env  RightPortType=workingframe  PhysicalDomain=Mechanical  DialogClass=GroundBlock  CoordPosition=[0 0 0]  CoordPositionUnits=cm  StateVectorMgrId=-1  MachineId=[0 0]  ShowEnvPort=on
  Engine Timer : Subsystem
  Friction : Subsystem
  Friction actuator : mblibv1/Sensors &  Actuators/Joint Actuator  Orientation=left  DialogController=MECH.DynMechDlgSource  SystemSampleTime=-1  PhysicalDomain=Mechanical  PortType=blob  ActuationStyle=Force  AngleUnits=deg  ArcVelocityUnits=deg/s  ArcAccelerationUnits=deg/s^2  CoordPositionUnits=m  VelocityUnits=m/s  AccelerationUnits=m/s^2  ForceUnits=N  TorqueUnits=N-m  ActiveIO=on  Width=1  DialogClass=MechanicalActuatorBlock  Primitive=R1  ReferenceFrame=Absolute (INERTIAL)
  Machine Environment : mblibv1/Bodies/Machine Environment  Tag=Factory ground  DialogController=MECH.DialogSource  SystemSampleTime=-1  PortType=env  PhysicalDomain=Mechanical  DialogTemplateClass=MECH.MachineEnvironment  SyncWhenCopied=off  Gravity=[0 -9.81 0]  GravityUnits=m/s^2  GravityAsSignal=off  Dimensionality=3D Only  AnalysisType=Forward dynamics  LinearAssemblyTolerance=1e-3  LinearAssemblyToleranceUnits=m  AngularAssemblyTolerance=1e-3  AngularAssemblyToleranceUnits=rad  ConstraintSolverType=Stabilizing  ConstraintRelTolerance=1e-4  ConstraintAbsTolerance=1e-4  UseRobustSingularityHandling=off  RedundancyAnalysisToleranceType=Automatically select tolerance  RedundancyAnalysisTolerance=1e-14  StatePerturbationType=Fixed  PerturbationSize=1e-5  VisualizeMachine=on
  Revolute : mblibv1/Joints/Revolute  DialogController=MECH.DynMechDlgSource  PhysicalDomain=mechanical  SubClassName=Unknown  LeftPortType=blob  RightPortType=blob  LConnTagsString=__newl0|SA1|SA2  RConnTagsString=__newr0|SA1  NumSAPorts=3  CutJoint=off  MarkAsCut=off  Primitives=revolute  PrimitiveProps=R1$WORLD$[1 0 0]$revolute  DialogClass=JointBlock  R1Axis=[1 0 0]
  Rod1 : PMIOPort  Orientation=down  Port=1  Side=Right
  Rod2 : PMIOPort  Orientation=down  Port=2  Side=Right
  Rod3 : PMIOPort  Orientation=down  Port=3  Side=Right
  Rod4 : PMIOPort  Orientation=down  Port=4  Side=Right
  Tacometer : PMIOPort  Port=5  Side=Left
  wires:
  Angle sensor/2 -> Friction/2(Rate)
  Friction/1(Torque) -> Friction actuator/1
  Angle sensor/1 -> Engine Timer/1(Angle), Friction/1(Angle)
  connections:
  Revolute/LConn2 -- Tacometer/RConn1
  Friction actuator/RConn1 -- Revolute/LConn3
  Revolute/RConn2 -- Angle sensor/LConn1
  Engine Block/RConn1 -- Revolute/LConn1
  Revolute/RConn1 -- Crank/LConn1
  Rod4/RConn1 -- Crank/RConn4
  Rod3/RConn1 -- Crank/RConn3
  Rod2/RConn1 -- Crank/RConn2
  Rod1/RConn1 -- Crank/RConn1
  Machine Environment/RConn1 -- Engine Block/LConn1

== system mech_fceng1/Stall ==
  "Fuel " : Inport  OutDataType=sfix(16)  OutScaling=2^0
  Gain1 : Gain  Orientation=down  Gain=0.05  ParameterDataType=sfix(16)  ParameterScaling=2^0  OutDataType=sfix(16)  OutScaling=2^0  SaturateOnIntegerOverflow=on  OutDataTypeStr=Inherit: Same as input  ParamDataTypeStr=Inherit: Same as input
  Gain2 : Gain  Orientation=down  Gain=-1  ParameterDataType=sfix(16)  ParameterScaling=2^0  OutDataType=sfix(16)  OutScaling=2^0  SaturateOnIntegerOverflow=on  OutDataTypeStr=Inherit: Same as input  ParamDataTypeStr=Inherit: Same as input
  Gain3 : Gain  Orientation=down  Gain=-1  ParameterDataType=sfix(16)  ParameterScaling=2^0  OutDataType=sfix(16)  OutScaling=2^0  SaturateOnIntegerOverflow=on  OutDataTypeStr=Inherit: Same as input  ParamDataTypeStr=Inherit: Same as input
  Mux : Mux  Orientation=down
  Switch : Switch  Orientation=down  Threshold=0.5  ZeroCross=off  InputSameDT=on
  Switch1 : Switch  Orientation=down  Threshold=0.5  ZeroCross=off  InputSameDT=on
  Fuel : Outport  Orientation=down  OutDataType=sfix(16)  OutScaling=2^0
  wires:
  "Fuel "/1 -> Gain1/1
  Switch/1 -> Mux/1
  Gain1/1 -> Mux/2, Mux/3, Switch/1, Switch1/1
  Switch1/1 -> Mux/4
  Mux/1 -> Fuel/1
  Gain2/1 -> Switch/2
  Gain3/1 -> Switch1/2
  [Cylinder1] -> Gain2/1
  [Cylinder2] -> Gain3/1

== system mech_fceng1/Tachometer ==
  note: RPM
  Constant : Constant  Value=0  OutDataType=sfix(16)  OutScaling=2^0
  Engine RPM : Scope
      settings: Tag=OpenMeAtStartUp  YMin=0  YMax=900  SaveName=ScopeData2
  Gain1 : Gain  Orientation=left  Gain=60/(2*pi)  ParameterDataType=sfix(16)  ParameterScaling=2^0  OutDataType=sfix(16)  OutScaling=2^0  SaturateOnIntegerOverflow=on  OutDataTypeStr=Inherit: Same as input  ParamDataTypeStr=Inherit: Same as input
  Joint Sensor : mblibv1/Sensors &  Actuators/Joint Sensor  Orientation=left  DialogController=MECH.DynMechDlgSource  SystemSampleTime=-1  PhysicalDomain=Mechanical  PortType=blob  Muxed=on  Pose=off  Angle=off  AngleUnits=deg  ArcVelocity=on  ArcVelocityUnits=rad/s  ArcAcceleration=off  ArcAccelerationUnits=deg/s^2  CoordPosition=on  CoordPositionUnits=m  Velocity=off  VelocityUnits=m/s  Acceleration=off  AccelerationUnits=m/s^2  Quaternion=on  QuaternionDT=off  QuaternionDDT=off  QuaternionUnits=off  OutputVector=[ 1 ]  ActiveIO=on  Width=1  DialogClass=MechanicalSensorBlock  Primitive=R1  Force=off  ForceUnits=N  Torque=off  TorqueUnits=N-m  ReferenceFrame=Absolute (INERTIAL)  ReactionSensedSide=Base  ReactionReferenceFrame=Absolute (World)  ReactionForce=off  ReactionForceUnits=N  ReactionMoment=off  ReactionMomentUnits=N-m
  Relational Operator : RelationalOperator  Operator=<  ZeroCross=off  InputSameDT=on
  Stop Simulation : Stop
  Transfer Fcn : TransferFcn  Orientation=left  Numerator=[15]  Denominator=[1 15]
  Rate : PMIOPort  Tag=PMCPort  Orientation=left  Port=1  Side=Left
  wires:
  Gain1/1 -> Relational Operator/1, Transfer Fcn/1
  Constant/1 -> Relational Operator/2
  Joint Sensor/1 -> Gain1/1
  Relational Operator/1 -> Stop Simulation/1
  Transfer Fcn/1 -> Engine RPM/1  "RPM"
  connections:
  Rate/RConn1 -- Joint Sensor/LConn1

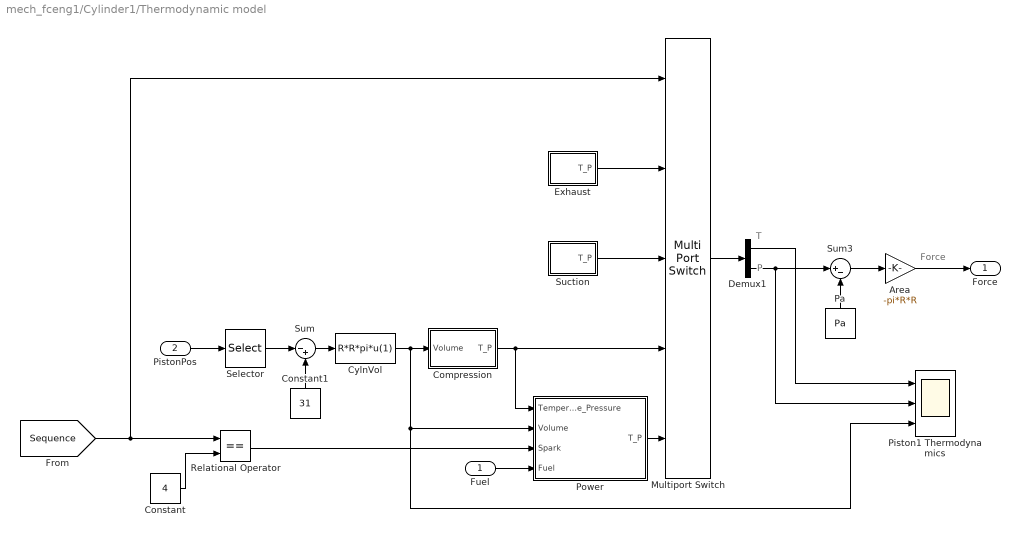
== system mech_fceng1/Cylinder1/Thermodynamic model ==
  note: Force
  note: P
  note: T
  Fuel : Inport  OutDataType=sfix(16)  OutScaling=2^0
  PistonPos : Inport  Port=2  OutDataType=sfix(16)  OutScaling=2^0
  Area : Gain  Gain=-pi*R*R  ParameterDataType=sfix(16)  ParameterScaling=2^0  OutDataType=sfix(16)  OutScaling=2^0  SaturateOnIntegerOverflow=on  OutDataTypeStr=Inherit: Same as input  ParamDataTypeStr=Inherit: Same as input
  Compression : Subsystem
  Constant : Constant  Value=4  OutDataType=sfix(16)  OutScaling=2^0
  Constant1 : Constant  Orientation=up  Value=31  OutDataType=sfix(16)  OutScaling=2^0
  CylnVol : Fcn  Expr=R*R*pi*u(1)
  Demux1 : Demux  Outputs=2
  Exhaust : Subsystem  TreatAsAtomicUnit=on
  Multiport Switch : MultiPortSwitch  Inputs=4  InputSameDT=on
  Pa : Constant  Orientation=up  Value=Pa  OutDataType=sfix(16)  OutScaling=2^0
  Piston1 Thermodynamics : Scope  NumInputPorts=3
      settings: YMin=25~0~50  YMax=425~240000~1050
  Power : Subsystem
  Relational Operator : RelationalOperator  Operator===  ZeroCross=off  InputSameDT=on
  Selector : Selector  InputPortWidth=3  IndexOptions=Index vector (dialog)  Indices=2  OutputSizes=1
  Suction : Subsystem  TreatAsAtomicUnit=on
  Sum : Sum  Inputs=|-+  OutDataType=sfix(16)  OutScaling=2^0  SaturateOnIntegerOverflow=on  InputSameDT=on  OutDataTypeStr=Inherit: Same as first input
  Sum3 : Sum  Inputs=|+-  OutDataType=sfix(16)  OutScaling=2^0  SaturateOnIntegerOverflow=on  InputSameDT=on  OutDataTypeStr=Inherit: Same as first input
  Force : Outport  OutDataType=sfix(16)  OutScaling=2^0
  wires:
  PistonPos/1 -> Selector/1
  Selector/1 -> Sum/1
  [Sequence] -> Multiport Switch/1, Relational Operator/1
  Relational Operator/1 -> Power/3(Spark)
  Area/1 -> Force/1
  Sum/1 -> CylnVol/1
  Constant/1 -> Relational Operator/2
  Demux1/1 -> Piston1 Thermodynamics/1
  Compression/1(T_P) -> Multiport Switch/4, Power/1(Temperature_Pressure)
  CylnVol/1 -> Piston1 Thermodynamics/3, Power/2(Volume), Compression/1(Volume)
  Constant1/1 -> Sum/2
  Fuel/1 -> Power/4(Fuel)
  Power/1(T_P) -> Multiport Switch/5
  Demux1/2 -> Piston1 Thermodynamics/2, Sum3/1
  Sum3/1 -> Area/1
  Pa/1 -> Sum3/2
  Multiport Switch/1 -> Demux1/1
  Exhaust/1(T_P) -> Multiport Switch/2
  Suction/1(T_P) -> Multiport Switch/3
